simulink model "Hadamard_Stream_Ex1"  (R2025a)
settings: Solver=VariableStepAuto  StartTime=0.0  StopTime=10  RelTol=1e-3
undefined symbols (not defined in the file): Correlation_ValidMode, DUT, L, vsva1596, xcvc1702
libraries: aieUtilities x4, aieDSP x1, vmcUtilities x1
settings Model: Creator=sdegala  LastModifiedBy=robg
settings ModelReferenceCC: EnableRefExpFcnMdlSchedulingChecks=on
settings RTWCC: GPUComputeCapability=3.5

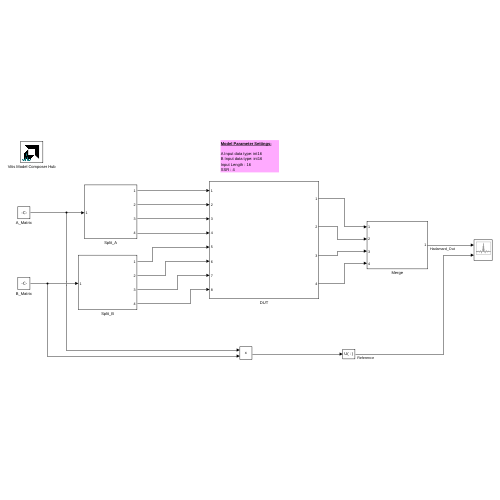
[thumbnail: Simulink's stored preview of the top-level diagram]
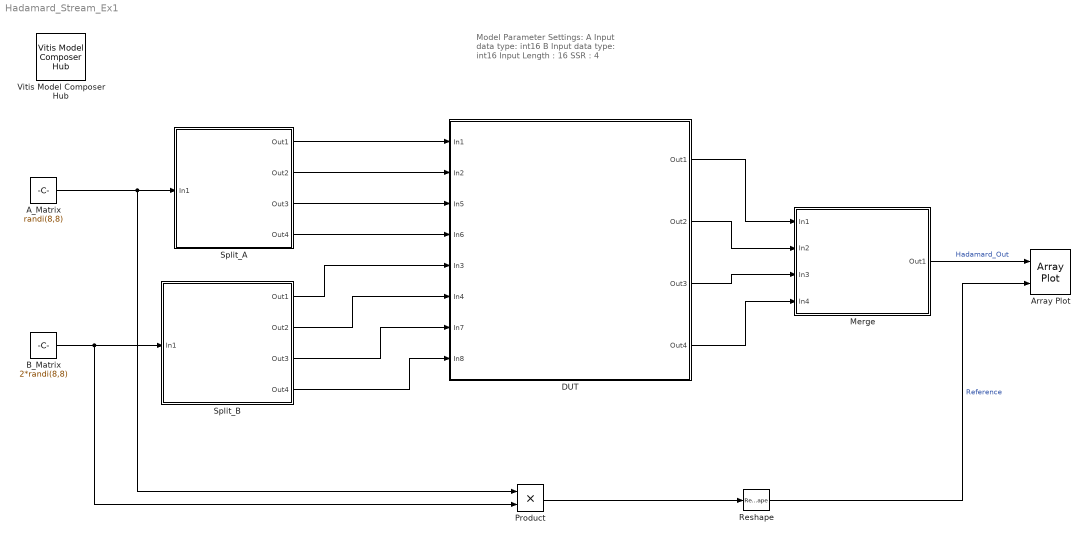
== system Hadamard_Stream_Ex1 ==
  note: Model Parameter Settings:
      |
      | A Input data type: int16
      | B Input data type: int16
      | Input Length : 16
      | SSR : 4
  A_Matrix : Constant  Value=randi(8,8)  OutDataTypeStr=int16  SampleTime=1
  Array Plot : ArrayPlot  NumInputPorts=2  WindowPosition=[270.000000,224.000000,800.000000,500.000000,]  Visible=on  ScopeFrameLocation=window  YLimits=[-11.75 125.75]  ShowLegend=on
  B_Matrix : Constant  Value=2*randi(8,8)  OutDataTypeStr=int16  SampleTime=1
  DUT : Subsystem
  Merge : Subsystem
  Product : Product
  Reshape : Reshape
  Split_A : Subsystem
  Split_B : Subsystem
  Vitis Model Composer Hub : vmcUtilities/Vitis Model Composer Hub  Tag=genX  CodeGeneration=off  SubsystemName=DUT  BlockHierPath=Correlation_ValidMode/DUT  SubsystemType=AIENode  StartColumn=1  NumberOfColumns=1  TargetDirectory=./code  exportDesign=off  analyzeDesign=on  validateDesignOnHw=off  ExportType=AI Engines  IpVendor=xilinx.com  IpLibrary=hls  IpVersion=1.0  IpHWLanguage=Verilog  AieCompilerOptions={}  AieSimulatorOptions={}  AieGraphIterations=-1  CreateTestbench=on  TestbenchStackSize=10  RunRtlSim=off  RunCSim=off  RunAieSim=off  AieSimTimeout=50000  RunAieSimProfiling=off  LaunchVitisAnalyzer=off  PlotOutput=off  RunX86Sim=off  X86SimTimeout=10  GenHwImage=off  GenLibadfXo=off  GenHwValidationCode=off  PlatformType=Not Specified  HwSystemType=Baremetal  HwValidationTarget=hw  ProjDevice=xcvc1702-vsva1596-2LP-e-L  ProjDevicePart=xcvc1702-vsva1596-2LP-e-L  AIEType=AIE  SamplePeriod=-1  ClockFrequency=200  DataPathParallelism=1  xilinxfamily=versalaicore  part=xcvc1702  speed=-2LP-e-L  package=vsva1596  directory=./netlist  testbench=off  incr_netlist=off  synthesis_tool=Vivado  clock_wrapper=Clock Enables  dbl_ovrd=According to Block Masks  dcm_input_clock_period=10  sysclk_period=10  simulink_period=1  eval_field=0  IPInfoJsonString="{\"DUTSubsystemName\":\"DUT\",\"AIESubsystem\":{\"SubsystemName\":\"DUT\",\"TargetDirectory\":\"./code\",\"AIEArrayConfig\":\"Use entire AIE array\",\"StartColumn\":\"0\",\"NumberOfColumns\":\"1\"},\"SubsystemTag\":\"AIENode\"}"  LogFileName=/proj/xhdhdstaff5/sdegala/Head1/HEAD/2025_2_work/AIE_BLOCKS_2025_2/code/model_composer.log  NThreads=4  IPConfigFile=/tmp/vmctmp-11198269997411262707/Correlation_ValidMode_ipconfig.json
  wires:
  DUT/1(Out1) -> Merge/1(In1)
  DUT/2(Out2) -> Merge/2(In2)
  Reshape/1 -> Array Plot/2  "Reference"
  Split_B/2(Out2) -> DUT/6(In4)
  Product/1 -> Reshape/1
  B_Matrix/1 -> Product/2, Split_B/1(In1)
  Merge/1(Out1) -> Array Plot/1  "Hadamard_Out"
  Split_A/1(Out1) -> DUT/1(In1)
  Split_A/2(Out2) -> DUT/2(In2)
  Split_B/1(Out1) -> DUT/5(In3)
  A_Matrix/1 -> Product/1, Split_A/1(In1)
  Split_A/3(Out3) -> DUT/3(In5)
  Split_A/4(Out4) -> DUT/4(In6)
  Split_B/3(Out3) -> DUT/7(In7)
  Split_B/4(Out4) -> DUT/8(In8)
  DUT/3(Out3) -> Merge/3(In3)
  DUT/4(Out4) -> Merge/4(In4)

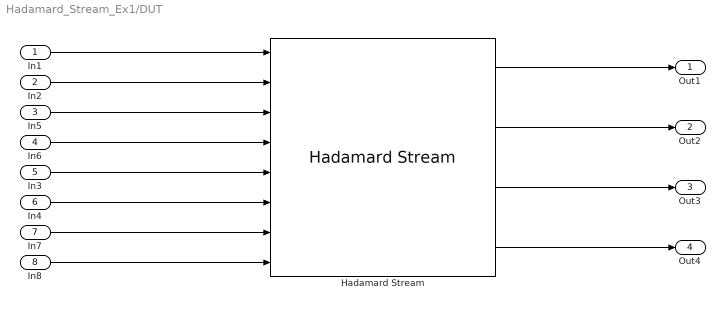
== system Hadamard_Stream_Ex1/DUT ==
  In1 : Inport
  In2 : Inport  Port=2
  In5 : Inport  Port=3
  In6 : Inport  Port=4
  In3 : Inport  Port=5
  In4 : Inport  Port=6
  In7 : Inport  Port=7
  In8 : Inport  Port=8
  Hadamard Stream : aieDSP/Hadamard Stream  AIE_VARIANT=1  TP_API=1  data_type_A=int16  data_type_B=int16  dim_size=64  num_frames=1  shift_output=0  ssr=4  rnd_mode=Floor  sat_mode=None  blockJsonConstraints=[]  blockJsonConstraintsInternal=[]  spec=vmc_stream_hadamard.json  SerializedMaskParamNames=[]  SerializedMaskParamValues=[]  SerializedMaskParamVisibilities=[]  block_type=Hadamard Stream  SerializedMaskParamDataypes=uint|uint|typename|typename|uint|uint|uint|uint|uint|uint  SerializedMaskParamEnumStrArr=0|0|0|0|0|0|0|0|Floor,Ceiling,Round to positive infinity,Round to negative infinity,Round symmetrical to infinity,Round symmetrical to zero,Round convergent to even,Round convergent to odd|None,Saturate,Symmetric  SerializedMaskParamEnumValArr=0|0|0|0|0|0|0|0|0,1,2,3,4,5,6,7|0,1,3  SerializedMaskParamVectorArr=0|0|0|0|0|0|0|0|0|0  SerializedMaskParamKeys=AIE_VARIANT|TP_API|TT_DATA_A|TT_DATA_B|TP_DIM|TP_NUM_FRAMES|TP_SHIFT|TP_SSR|TP_RND|TP_SAT
  Out1 : Outport
  Out2 : Outport  Port=2
  Out3 : Outport  Port=3
  Out4 : Outport  Port=4
  wires:
  In1/1 -> Hadamard Stream/1
  In2/1 -> Hadamard Stream/2
  Hadamard Stream/2 -> Out2/1
  In4/1 -> Hadamard Stream/6
  Hadamard Stream/1 -> Out1/1
  In3/1 -> Hadamard Stream/5
  In5/1 -> Hadamard Stream/3
  In6/1 -> Hadamard Stream/4
  In8/1 -> Hadamard Stream/8
  In7/1 -> Hadamard Stream/7
  Hadamard Stream/4 -> Out4/1
  Hadamard Stream/3 -> Out3/1

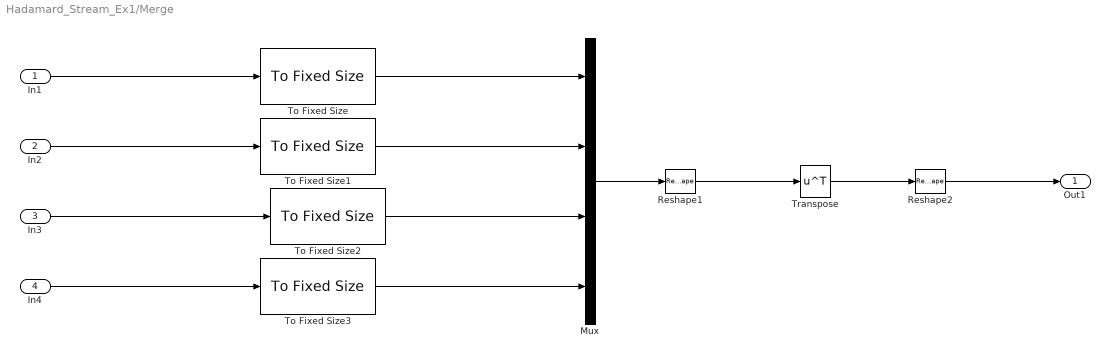
== system Hadamard_Stream_Ex1/Merge ==
  In1 : Inport
  In2 : Inport  Port=2
  In3 : Inport  Port=3
  In4 : Inport  Port=4
  Mux : Mux
  Reshape1 : Reshape  OutputDimensionality=Customize  OutputDimensions=[16, 4]
  Reshape2 : Reshape  OutputDimensions=[1, 10]
  To Fixed Size{,1..3} (4 alike) : aieUtilities/To Fixed Size  Mode=Stop simulation when input variable-size signal is not full  OutputSize=Inherit: Same as input  CopyMethod=Buffer samples to form output  HasStatusOutput=on
  Transpose : Math  Operator=transpose
  Out1 : Outport
  wires:
  Reshape1/1 -> Transpose/1
  To Fixed Size/1 -> Mux/1
  In1/1 -> To Fixed Size/1
  In2/1 -> To Fixed Size1/1
  Transpose/1 -> Reshape2/1
  To Fixed Size1/1 -> Mux/2
  Reshape2/1 -> Out1/1
  Mux/1 -> Reshape1/1
  To Fixed Size2/1 -> Mux/3
  In4/1 -> To Fixed Size3/1
  In3/1 -> To Fixed Size2/1
  To Fixed Size3/1 -> Mux/4

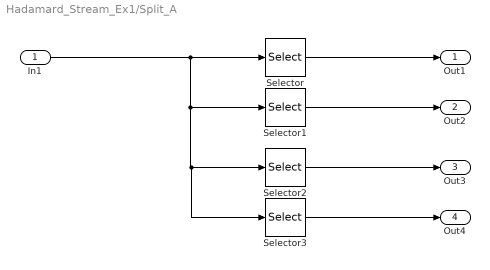
== system Hadamard_Stream_Ex1/Split_A ==
  In1 : Inport
  Selector : Selector  NumberOfDimensions=2  InputPortWidth=64  IndexOptions=Index vector (dialog),Index vector (dialog)  Indices=1:4:8,1:8  OutputSizes=1,1
  Selector1 : Selector  NumberOfDimensions=2  InputPortWidth=64  IndexOptions=Index vector (dialog),Index vector (dialog)  Indices=2:4:8,1:8  OutputSizes=1,1
  Selector2 : Selector  NumberOfDimensions=2  InputPortWidth=64  IndexOptions=Index vector (dialog),Index vector (dialog)  Indices=3:4:8,1:8  OutputSizes=1,1
  Selector3 : Selector  NumberOfDimensions=2  InputPortWidth=64  IndexOptions=Index vector (dialog),Index vector (dialog)  Indices=4:4:8,1:8  OutputSizes=1,1
  Out1 : Outport
  Out2 : Outport  Port=2
  Out3 : Outport  Port=3
  Out4 : Outport  Port=4
  wires:
  Selector1/1 -> Out2/1
  Selector/1 -> Out1/1
  Selector2/1 -> Out3/1
  Selector3/1 -> Out4/1
  In1/1 -> Selector/1, Selector3/1, Selector2/1, Selector1/1

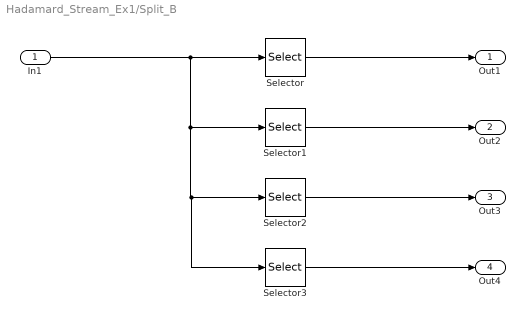
== system Hadamard_Stream_Ex1/Split_B ==
  In1 : Inport
  Selector : Selector  NumberOfDimensions=2  InputPortWidth=64  IndexOptions=Index vector (dialog),Index vector (dialog)  Indices=1:4:8,1:8  OutputSizes=1,1
  Selector1 : Selector  NumberOfDimensions=2  InputPortWidth=64  IndexOptions=Index vector (dialog),Index vector (dialog)  Indices=2:4:8,1:8  OutputSizes=1,1
  Selector2 : Selector  NumberOfDimensions=2  InputPortWidth=64  IndexOptions=Index vector (dialog),Index vector (dialog)  Indices=3:4:8,1:8  OutputSizes=1,1
  Selector3 : Selector  NumberOfDimensions=2  InputPortWidth=64  IndexOptions=Index vector (dialog),Index vector (dialog)  Indices=4:4:8,1:8  OutputSizes=1,1
  Out1 : Outport
  Out2 : Outport  Port=2
  Out3 : Outport  Port=3
  Out4 : Outport  Port=4
  wires:
  Selector1/1 -> Out2/1
  Selector/1 -> Out1/1
  Selector2/1 -> Out3/1
  Selector3/1 -> Out4/1
  In1/1 -> Selector/1, Selector3/1, Selector2/1, Selector1/1
